simulink model "chap2_1sim"  (R2023b)
settings: Solver=ode45  StartTime=0.0  StopTime=500  RelTol=1e-3
settings Model: Creator=CorgiQvm  LastModifiedBy=CorgiQvm
settings DataIOCC: LimitDataPoints=on  SaveFormat=Array  ReturnWorkspaceOutputs=off

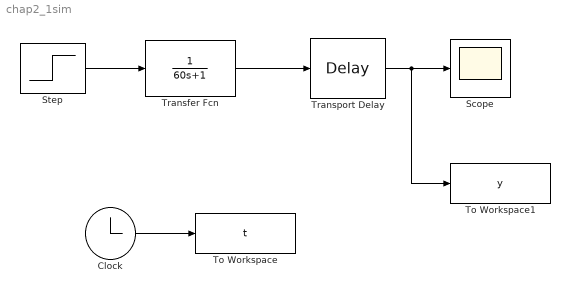
== system chap2_1sim ==
  Clock : Clock
  Scope : Scope
  Step : Step  Time=0  SampleTime=0
  To Workspace : ToWorkspace  VariableName=t  SampleTime=-1
  To Workspace1 : ToWorkspace  VariableName=y  SampleTime=-1
  Transfer Fcn : TransferFcn  Denominator=[60 1]
  Transport Delay : TransportDelay  DelayTime=80
  wires:
  Step/1 -> Transfer Fcn/1
  Transfer Fcn/1 -> Transport Delay/1
  Transport Delay/1 -> To Workspace1/1, Scope/1
  Clock/1 -> To Workspace/1
